simulink model "powerwindow05"  (Simulink 6.0)
settings: Solver=ode23t  StartTime=0.0  StopTime=inf  FixedStep=1e-4  RelTol=1e-2
InitFcn:
  | powericon('psbinitsys',bdroot);
libraries: powerlib x44, mblibv1 x18, simulink x8, dspquant2 x5, xpclib x4
(part 2 of 2)

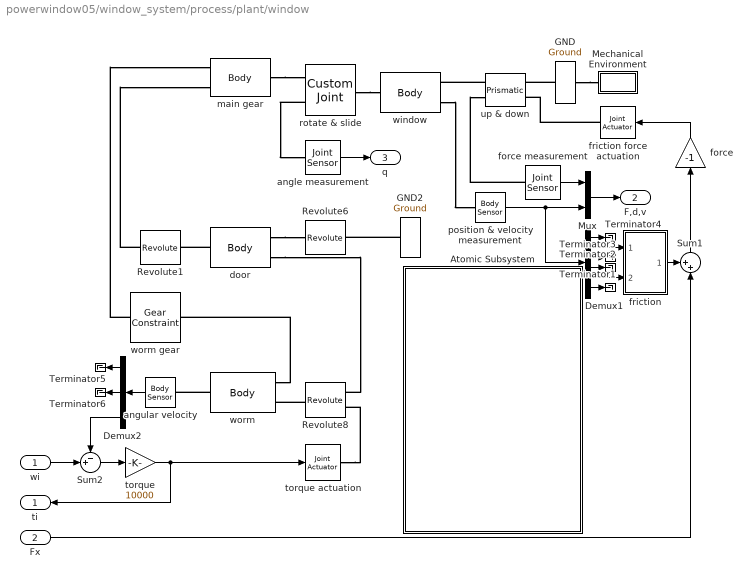
== system powerwindow05/window_system/process/plant/window ==
  wi : Inport  Port=1  LatchInput=off
  Fx : Inport  Port=2  LatchInput=off
  Atomic Subsystem : Subsystem  TreatAsAtomicUnit=on  PropExecContextAcrossSSBoundary=on
      mask Display: image(imread('pw_window1c.jpg'))
  Demux1 : Demux  Outputs=6
  Demux2 : Demux  Orientation=left  Outputs=3
  GND : mblibv1/Bodies/Ground  Orientation=left  Opaque=on  LeftPortType=env  RightPortType=workingframe  PhysicalDomain=Mechanical  DialogClass=GroundBlock  CoordPosition=[10 0 0]  CoordPositionUnits=cm  StateVectorMgrId=-1  MachineId=[0 0]  ShowEnvPort=on
  GND2 : mblibv1/Bodies/Ground  Orientation=left  Opaque=on  LeftPortType=env  RightPortType=workingframe  PhysicalDomain=Mechanical  DialogClass=GroundBlock  CoordPosition=[0 0 0]  CoordPositionUnits=m  StateVectorMgrId=-1  MachineId=[0 0]  ShowEnvPort=off
  Mechanical Environment : Subsystem  Tag=Factory ground  Orientation=left  DialogController=MECH.DialogSource  PropExecContextAcrossSSBoundary=on  Opaque=on  mask(Mechanical){PortType=env, PhysicalDomain=Mechanical, ClassName=Environment, DialogTemplateClass=MECH.MachineEnvironment, SyncWhenCopied=off, Gravity=[0 0 0], GravityUnits=m/s^2, GravityAsSignal=off, Dimensionality=3D Only, AnalysisType=Forward dynamics, LinearAssemblyTolerance=1e-3, LinearAssemblyToleranceUnits=m, AngularAssemblyTolerance=1e-3, AngularAssemblyToleranceUnits=rad, ConstraintSolverType=Stabilizing, ConstraintRelTolerance=1e-4, ConstraintAbsTolerance=1e-4, UseRobustSingularityHandling=off, StatePerturbationType=Fixed, PerturbationSize=1e-5, VisualizeMachine=on}
      mask help: Defines the mechanical simulation environment for the machine to which the block is connected: gravity, dimensionality, analysis mode, constraint solver type, tolerances, linearization, and visualization.
      mask init:
      | mech_environment_block('MaskInitialization', gcbh);
      settings: CopyFcn=mech_environment_block('CopyFcn', gcbh);
      mask Help: web(mech_help('environment'))
      mask StyleString: edit,edit,edit,edit,edit,edit,popup(km/s^2|m/s^2|cm/s^2|mm/s^2|mi/s^2|ft/s^2|in/s^2),checkbox,popup(2D Only|3D Only|Auto-detect),popup(Forward dynamics|Inverse dynamics|Kinematics|Trimming),edit,popup(km|m|cm|mm|mi|ft|in),edit,popup(deg|rad),popup(Stabilizing|Tolerancing|Machine precision),edit,edit,checkbox,popup(Adaptive|Fixed),edit,checkbox
      mask Display: disp('Env')
  Mux : Mux  Inputs=2
  Revolute1 : mblibv1/Joints/Revolute  Tag=Factory generic  Description=Mechanical Blockset  Orientation=left  PhysicalDomain=mechanical  SubClassName=Unknown  LeftPortType=blob  RightPortType=blob  LConnTagsString=__newl0  RConnTagsString=__newr0  NumSAPorts=0  CutJoint=off  MarkAsCut=off  Primitives=revolute  PrimitiveProps=R1$WORLD$[0 0 1]$revolute  DialogClass=JointBlock
  Revolute6 : mblibv1/Joints/Revolute  Tag=Factory generic  Description=Mechanical Blockset  Orientation=left  PhysicalDomain=mechanical  SubClassName=Unknown  LeftPortType=blob  RightPortType=blob  LConnTagsString=__newl0  RConnTagsString=__newr0  NumSAPorts=0  CutJoint=off  MarkAsCut=off  Primitives=revolute  PrimitiveProps=R1$WORLD$[1 0 0]$revolute  DialogClass=JointBlock
  Revolute8 : mblibv1/Joints/Revolute  Tag=Factory generic  Description=Mechanical Blockset  Orientation=left  PhysicalDomain=mechanical  SubClassName=Unknown  LeftPortType=blob  RightPortType=blob  LConnTagsString=__newl0|SA1  RConnTagsString=__newr0  NumSAPorts=1  CutJoint=off  MarkAsCut=off  Primitives=revolute  PrimitiveProps=R1$WORLD$[0 0 1]$revolute  DialogClass=JointBlock
  Sum1 : Sum  Orientation=up  Inputs=++|  SaturateOnIntegerOverflow=on  InputSameDT=on
  Sum2 : Sum  Inputs=-+|  SaturateOnIntegerOverflow=on  InputSameDT=on
  Terminator{1..6} (6 alike) : Terminator
  angle measurement : mblibv1/Sensors &  Actuators/Joint Sensor  Description=Mechanical Blockset  Opaque=on  PhysicalDomain=Mechanical  PortType=blob  Muxed=on  Pose=off  Angle=on  AngleUnits=rad  ArcVelocity=off  ArcVelocityUnits=deg/s  ArcAcceleration=off  ArcAccelerationUnits=deg/s^2  CoordPosition=off  CoordPositionUnits=m  Velocity=off  VelocityUnits=m/s  Acceleration=off  AccelerationUnits=m/s^2  Quaternion=on  QuaternionDT=off  QuaternionDDT=off  QuaternionUnits=off  OutputVector=[ 1 ]  ActiveIO=off  Width=1  DialogClass=MechanicalSensorBlock  Primitive=R1  Force=off  ForceUnits=N  Torque=off  TorqueUnits=N-m  ReferenceFrame=Absolute (INERTIAL)  ReactionSensedSide=Base  ReactionReferenceFrame=Absolute (World)  ReactionForce=off  ReactionForceUnits=N  ReactionMoment=off  ReactionMomentUnits=N-m
  angular velocity : mblibv1/Sensors &  Actuators/Body Sensor  Description=Mechanical Blockset  Orientation=left  Opaque=on  PhysicalDomain=Mechanical  PortType=blob  Muxed=on  Pose=off  Angle=on  AngleUnits=deg  ArcVelocity=on  ArcVelocityUnits=rad/s  ArcAcceleration=off  ArcAccelerationUnits=deg/s^2  CoordPosition=off  CoordPositionUnits=m  Velocity=off  VelocityUnits=m/s  Acceleration=off  AccelerationUnits=m/s^2  Quaternion=on  QuaternionDT=off  QuaternionDDT=off  QuaternionUnits=off  OutputVector=[ 3 ]  ActiveIO=off  Width=3  DialogClass=MechanicalSensorBlock  ReferenceFrame=Absolute (World)
  door : mblibv1/Bodies/Body  Tag=Factory generic  Description=Mechanical Blockset  Orientation=left  PhysicalDomain=mechanical  SubClassName=Unknown  LeftPortType=workingframe  RightPortType=workingframe  LConnTagsString=CS3|CG  RConnTagsString=CS1  DialogClass=MechanicalBodyBlock  Mass=1  MassUnits=kg  InertiaUnits=kg*m^2  Inertia=eye(3)  Shape=Cylinder  ShapeDims=[1 1]  ShapeUnits=m  ShapeUse=false  Density=1  DensityUnits=kg/m^3  DensityUse=false  CG=Left$CG$[0 0 0]$WORLD$WORLD$cm$[0 0 0]$Euler X-Y-Z$deg$WORLD$true  WorkingFrames=Left$CS3$[0 0 0]$CG$CG$cm$[0 0 0]$Euler X-Y-Z$deg$WORLD$true#Right$CS1$[17 0 0]$CG$CG$cm$[0 0 0]$Euler X-Y-Z$deg$WORLD$true
  force : Gain  Orientation=up  Gain=-1  SaturateOnIntegerOverflow=on
  force measurement : mblibv1/Sensors &  Actuators/Joint Sensor  Description=Mechanical Blockset  Opaque=on  PhysicalDomain=Mechanical  PortType=blob  Muxed=on  Pose=off  Angle=on  AngleUnits=deg  ArcVelocity=off  ArcVelocityUnits=deg/s  ArcAcceleration=off  ArcAccelerationUnits=deg/s^2  CoordPosition=off  CoordPositionUnits=m  Velocity=off  VelocityUnits=m/s  Acceleration=off  AccelerationUnits=m/s^2  Quaternion=on  QuaternionDT=off  QuaternionDDT=off  QuaternionUnits=off  OutputVector=[ 3 ]  ActiveIO=off  Width=3  DialogClass=MechanicalSensorBlock  Primitive=P1  Force=off  ForceUnits=N  Torque=off  TorqueUnits=N-m  ReferenceFrame=Absolute (INERTIAL)  ReactionSensedSide=Base  ReactionReferenceFrame=Absolute (World)  ReactionForce=on  ReactionForceUnits=N  ReactionMoment=off  ReactionMomentUnits=N-m
  friction : Subsystem  PropExecContextAcrossSSBoundary=on
  friction force actuation : mblibv1/Sensors &  Actuators/Joint Actuator  Description=Mechanical Blockset  Orientation=left  Opaque=on  PhysicalDomain=Mechanical  PortType=blob  ActuationStyle=Force  AngleUnits=deg  ArcVelocityUnits=deg/s  ArcAccelerationUnits=deg/s^2  CoordPositionUnits=m  VelocityUnits=m/s  AccelerationUnits=m/s^2  ForceUnits=N  TorqueUnits=N-m  ActiveIO=off  Width=1  DialogClass=MechanicalActuatorBlock  Primitive=P1  ReferenceFrame=Absolute (INERTIAL)
  main gear : mblibv1/Bodies/Body  Tag=Factory generic  Description=Mechanical Blockset  PhysicalDomain=mechanical  SubClassName=Unknown  LeftPortType=workingframe  RightPortType=workingframe  LConnTagsString=CS3|CG  RConnTagsString=CS1  DialogClass=MechanicalBodyBlock  Mass=2  MassUnits=kg  InertiaUnits=kg*m^2  Inertia=eye(3)  Shape=Cylinder  ShapeDims=[1 1]  ShapeUnits=m  ShapeUse=false  Density=1  DensityUnits=kg/m^3  DensityUse=false  CG=Left$CG$[17 0 0]$WORLD$WORLD$cm$[0 0 0]$Euler X-Y-Z$deg$WORLD$true  WorkingFrames=Left$CS3$[0 0 0]$CG$CG$cm$[0 0 0]$Euler X-Y-Z$deg$WORLD$true#Right$CS1$[60 0 0]$CG$CG$cm$[0 0 0]$Euler X-Y-Z$deg$WORLD$true
  position & velocity measurement : mblibv1/Sensors &  Actuators/Body Sensor  Description=Mechanical Blockset  Opaque=on  PhysicalDomain=Mechanical  PortType=blob  Muxed=on  Pose=off  Angle=on  AngleUnits=deg  ArcVelocity=off  ArcVelocityUnits=deg/s  ArcAcceleration=off  ArcAccelerationUnits=deg/s^2  CoordPosition=on  CoordPositionUnits=m  Velocity=on  VelocityUnits=m/s  Acceleration=off  AccelerationUnits=m/s^2  Quaternion=on  QuaternionDT=off  QuaternionDDT=off  QuaternionUnits=off  OutputVector=[ 3 3 ]  ActiveIO=off  Width=6  DialogClass=MechanicalSensorBlock  ReferenceFrame=Absolute (World)
  rotate & slide : mblibv1/Joints/Custom Joint  Tag=Factory generic  Description=Mechanical Blockset  PhysicalDomain=mechanical  SubClassName=custom_joint  LeftPortType=blob  RightPortType=blob  LConnTagsString=__newl0|SA1  RConnTagsString=__newr0  NumSAPorts=1  CutJoint=off  MarkAsCut=off  Primitives=revolute_prismatic  PrimitiveProps=R1$Base$[0 0 1]$revolute#P1$Follower$[1 0 0]$prismatic  DialogClass=JointBlock
  torque : Gain  Gain=10000  SaturateOnIntegerOverflow=on
  torque actuation : mblibv1/Sensors &  Actuators/Joint Actuator  Description=Mechanical Blockset  Opaque=on  PhysicalDomain=Mechanical  PortType=blob  ActuationStyle=Force  AngleUnits=deg  ArcVelocityUnits=deg/s  ArcAccelerationUnits=deg/s^2  CoordPositionUnits=m  VelocityUnits=m/s  AccelerationUnits=m/s^2  ForceUnits=N  TorqueUnits=N-m  ActiveIO=off  Width=1  DialogClass=MechanicalActuatorBlock  Primitive=R1  ReferenceFrame=Absolute (INERTIAL)
  up & down : mblibv1/Joints/Prismatic  Tag=Factory generic  Description=Mechanical Blockset  Orientation=left  PhysicalDomain=mechanical  SubClassName=Unknown  LeftPortType=blob  RightPortType=blob  LConnTagsString=__newl0|SA1  RConnTagsString=__newr0|SA1  NumSAPorts=2  CutJoint=on  MarkAsCut=off  Primitives=prismatic  PrimitiveProps=P1$WORLD$[0 1 0]$prismatic  DialogClass=JointBlock
  window : mblibv1/Bodies/Body  Tag=Factory generic  Description=Mechanical Blockset  PhysicalDomain=mechanical  SubClassName=Unknown  LeftPortType=workingframe  RightPortType=workingframe  LConnTagsString=CS1  RConnTagsString=CS2|CS3  DialogClass=MechanicalBodyBlock  Mass=5  MassUnits=kg  InertiaUnits=kg*m^2  Inertia=eye(3)  Shape=Cylinder  ShapeDims=[1 1]  ShapeUnits=m  ShapeUse=false  Density=1  DensityUnits=kg/m^3  DensityUse=false  CG=Left$CG$[10 0 0]$WORLD$WORLD$cm$[0 0 0]$Euler X-Y-Z$deg$WORLD$false  WorkingFrames=Left$CS1$[0 0 0]$CG$CG$cm$[0 0 0]$Euler X-Y-Z$deg$WORLD$true#Right$CS2$[0 0 0]$CG$CG$cm$[0 0 0]$Euler X-Y-Z$deg$WORLD$true#Right$CS3$[-15 0 0]$CG$CG$cm$[0 0 0]$Euler X-Y-Z$deg$WORLD$true
  worm : mblibv1/Bodies/Body  Tag=Factory generic  Description=Mechanical Blockset  Orientation=left  PhysicalDomain=mechanical  SubClassName=Unknown  LeftPortType=workingframe  RightPortType=workingframe  LConnTagsString=CS3|CS4  RConnTagsString=CG  DialogClass=MechanicalBodyBlock  Mass=0.5  MassUnits=kg  InertiaUnits=kg*m^2  Inertia=eye(3)  Shape=Cylinder  ShapeDims=[1 1]  ShapeUnits=m  ShapeUse=false  Density=1  DensityUnits=kg/m^3  DensityUse=false  CG=Right$CG$[0 0 0]$WORLD$WORLD$cm$[0 0 0]$Euler X-Y-Z$deg$WORLD$true  WorkingFrames=Left$CS3$[0 0 0]$CG$CG$cm$[0 0 0]$Euler X-Y-Z$deg$WORLD$true#Left$CS4$[0 0 0]$CG$CG$cm$[0 0 0]$Euler X-Y-Z$deg$WORLD$true
  worm gear : mblibv1/Constraints &  Drivers/Gear Constraint  Tag=Factory generic  Description=Mechanical Blockset  Orientation=left  PhysicalDomain=mechanical  SubClassName=Unknown  LeftPortType=blob  RightPortType=blob  LConnTagsString=__newl0  RConnTagsString=__newr0  DialogClass=GearConstraint  NumSAPorts=0  BaseRadius=2  BaseRadiusUnits=cm  FollowerRadius=15  FollowerRadiusUnits=cm
  ti : Outport  Orientation=left
  F,d,v : Outport  Port=2
  q : Outport  Port=3
  wires:
  angle measurement/1 -> q/1
  Mux/1 -> F,d,v/1
  force measurement/1 -> Mux/1
  position & velocity measurement/1 -> Mux/2, Demux1/1
  Demux1/2 -> friction/1(position)
  Demux1/5 -> friction/2(velocity)
  torque/1 -> ti/1, torque actuation/1
  Sum2/1 -> torque/1
  angular velocity/1 -> Demux2/1
  Demux2/3 -> Sum2/1
  wi/1 -> Sum2/2
  Fx/1 -> Sum1/2
  friction/1(torque) -> Sum1/1
  Sum1/1 -> force/1
  force/1 -> friction force actuation/1
  Demux1/6 -> Terminator1/1
  Demux1/4 -> Terminator2/1
  Demux1/3 -> Terminator3/1
  Demux1/1 -> Terminator4/1
  Demux2/1 -> Terminator5/1
  Demux2/2 -> Terminator6/1
  connections:
  rotate & slide/LConn2 -- angle measurement/LConn1
  force measurement/LConn1 -- up & down/RConn2
  friction force actuation/RConn1 -- up & down/LConn2
  Revolute8/RConn1 -- worm/LConn2
  worm/LConn1 -- worm gear/LConn1
  door/RConn1 -- Revolute1/LConn1
  Revolute1/RConn1 -- main gear/LConn2
  worm gear/RConn1 -- main gear/LConn1
  door/LConn1 -- Revolute6/RConn1
  GND2/RConn1 -- Revolute6/LConn1
  torque actuation/RConn1 -- Revolute8/LConn2
  door/LConn2 -- Revolute8/LConn1
  main gear/RConn1 -- rotate & slide/LConn1
  rotate & slide/RConn1 -- window/LConn1
  window/RConn2 -- position & velocity measurement/LConn1
  GND/RConn1 -- up & down/LConn1
  up & down/RConn1 -- window/RConn1
  worm/RConn1 -- angular velocity/LConn1
  GND/LConn1 -- Mechanical Environment/RConn1

== system powerwindow05/window_system/process/plant/window/Atomic Subsystem ==

== system powerwindow05/window_system/process/plant/window/Mechanical Environment ==
  SOURCE_BLOCK : Constant  Value=Gravity
  TERM_BLOCK : Terminator
  out : PMIOPort  Port=1  Side=Right
  tag scope: sim_mech_tagd5028cb2b8530a0d=global
  wires:
  [sim_mech_tagd5028cb2b8530a0d] -> TERM_BLOCK/1
  SOURCE_BLOCK/1 -> [sim_mech_tagd5028cb2b8530a0d]

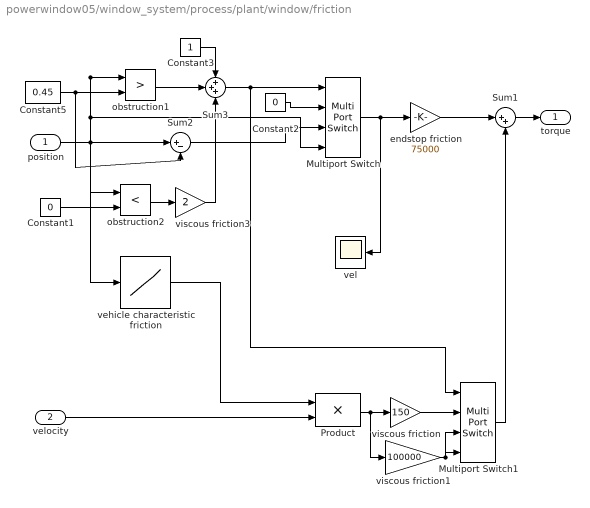
== system powerwindow05/window_system/process/plant/window/friction ==
  position : Inport  Port=1  LatchInput=off
  velocity : Inport  Port=2  LatchInput=off
  Constant1 : Constant  Value=0
  Constant2 : Constant  Value=0
  Constant3 : Constant
  Constant5 : Constant  Value=0.45
  Multiport Switch : MultiPortSwitch  Inputs=3  InputSameDT=on
  Multiport Switch1 : MultiPortSwitch  Inputs=3  InputSameDT=on
  Product : Product  SaturateOnIntegerOverflow=on  InputSameDT=on
  Sum1 : Sum  Inputs=|++  SaturateOnIntegerOverflow=on  InputSameDT=on
  Sum2 : Sum  Inputs=|+-  SaturateOnIntegerOverflow=on  InputSameDT=on
  Sum3 : Sum  Inputs=+++  SaturateOnIntegerOverflow=on  InputSameDT=on
  endstop friction : Gain  Gain=75000  SaturateOnIntegerOverflow=on
  obstruction1 : RelationalOperator  Operator=>  InputSameDT=on
  obstruction2 : RelationalOperator  Operator=<  InputSameDT=on
  vehicle characteristic friction : Lookup  DialogController=Simulink.DDGSource  InputValues=[0 2.5 10 11.5 14 24 30 31 35 47 50]  OutputValues=[1.15 1.2 1.05 1.1 1.05 1 1.1 1 0.95 0.9 0.95]  SaturateOnIntegerOverflow=on
  vel : Scope
      settings: YMin=-1  YMax=1  SaveName=ScopeData6
  viscous friction3 : Gain  Gain=2  SaturateOnIntegerOverflow=on
  viscous friction : Gain  Gain=150  SaturateOnIntegerOverflow=on
  viscous friction1 : Gain  Gain=100000  SaturateOnIntegerOverflow=on
  torque : Outport
  wires:
  Sum1/1 -> torque/1
  velocity/1 -> Product/2
  position/1 -> obstruction1/1, obstruction2/1, Multiport Switch/4, Sum2/1, vehicle characteristic friction/1
  Constant5/1 -> obstruction1/2, Sum2/2
  Constant1/1 -> obstruction2/2
  endstop friction/1 -> Sum1/1
  Constant2/1 -> Multiport Switch/2
  Sum2/1 -> Multiport Switch/3
  obstruction2/1 -> viscous friction3/1
  obstruction1/1 -> Sum3/2
  viscous friction3/1 -> Sum3/3
  Constant3/1 -> Sum3/1
  Sum3/1 -> Multiport Switch/1, Multiport Switch1/1
  Multiport Switch/1 -> endstop friction/1, vel/1
  Product/1 -> viscous friction/1, viscous friction1/1
  vehicle characteristic friction/1 -> Product/1
  viscous friction/1 -> Multiport Switch1/2
  Multiport Switch1/1 -> Sum1/2
  viscous friction1/1 -> Multiport Switch1/3, Multiport Switch1/4

== stateflow chart power_window_control_system/control ==
  settings: executeAtInitialization=1
  state emergencyDown
    entry:
    moveUp = 0;
    moveDown = 1;
  state safe
    state driverUp
      entry: moveUp = 1;
      exit: moveUp = 0;
      state iniDriverUp
      state DriverUp
      state autoDriverUp
      iniDriverUp -> (junction 26) : after(100,ticks)
      (junction 26) -> DriverUp
      (junction 26) -> autoDriverUp : [driver[1]]
    state driverDown
      entry: moveDown = 1;
      exit: moveDown = 0;
      state iniDriverDown
      state DriverDown
      state autoDriverDown
      iniDriverDown -> (junction 25) : after(100,ticks)
      (junction 25) -> autoDriverDown : [driver[1]]
      (junction 25) -> DriverDown
    state driverNeutral
      entry:
      moveUp = 0;
      moveDown = 0;
      state passengerneutral
        entry:
        moveUp = 0;
        moveDown = 0;
      state passengerUp
        entry: moveUp = 1;
        exit: moveUp = 0;
        state iniPassengerUp
        state PassengerUp
        state autoPassengerUp
        (junction 24) -> PassengerUp
        (junction 24) -> autoPassengerUp : [passenger[1]]
        iniPassengerUp -> (junction 24) : after(100,ticks)
      state passengerDown
        entry: moveDown = 1;
        exit: moveDown = 0;
        state iniPassengerDown
        state passengerDown
        state autoPassengerDown
        (junction 23) -> autoPassengerDown : [passenger[1]]
        iniPassengerDown -> (junction 23) : after(100,ticks)
        (junction 23) -> safe.driverNeutral.passengerDown.passengerDown
      safe.driverNeutral.passengerDown.passengerDown -> passengerneutral : [passenger[1]]
      safe.driverNeutral.passengerDown -> passengerneutral : [endstop]
      PassengerUp -> passengerneutral : [passenger[1]]
      passengerUp -> passengerneutral : [endstop]
      passengerneutral -> iniPassengerDown : [passenger[3]]
      passengerneutral -> iniPassengerUp : [passenger[2]]
      safe.driverNeutral.passengerDown -> PassengerUp : [passenger[2]]
      passengerUp -> safe.driverNeutral.passengerDown.passengerDown : [passenger[3]]
      (default) -> passengerneutral
    driverNeutral -> iniDriverDown : [driver[3]]
    driverUp -> DriverDown : [driver[3]]
    driverDown -> DriverUp : [driver[2]]
    driverNeutral -> iniDriverUp : [driver[2]]
    DriverDown -> driverNeutral : [driver[1]]
    DriverUp -> driverNeutral : [driver[1]]
    driverDown -> driverNeutral : [endstop]
    driverUp -> driverNeutral : [endstop]
    (default) -> driverNeutral
  emergencyDown -> passengerneutral : [endstop | after(100,ticks)]
  safe -> emergencyDown : [obstacle]
  (default) -> safe
  data: moveUp output double size=1; moveDown output double size=1; endstop input boolean size=1; obstacle input boolean size=1; driver input boolean size=3; passenger input boolean size=3
  events: ticks input EITHER_EDGE_EVENT

== stateflow chart power_window_control_system/detect_obstacle_endstop/detect_obstacle/delay_detection ==
  settings: executeAtInitialization=1
  state detect
  state off
  state hold
  (default) -> off
  off -> hold : [move_up]
  detect -> off : [~move_up]
  hold -> detect : [after(100,ticks)]
  hold -> off : [~move_up]
  data: detect output State size=1; move_up input boolean size=1
  events: ticks input EITHER_EDGE_EVENT
